simulink model "lowpasscont2"  (Simulink 8.3)
settings: Solver=ode4  StartTime=0.0  StopTime=10.24  FixedStep=dt  MaxStep=自動  MinStep=自動  RelTol=1e-3  AbsTol=自動
values from neighbouring files (symbols this model uses):
  dt = 0.01    [p217.m]    (also in p218_2.m; p223.m)
settings Model: Creator=ikko  LastModifiedBy=ikko
settings SolverCC: InitialStep=自動
settings DataIOCC: SignalLoggingName=logsOut
settings OptimizationCC: ExpressionDepthLimit=2147483647  InitFltsAndDblsToZero=on
settings DebuggingCC: SaveWithParameterizedLinksMsg=none  CheckExecutionContextPreStartOutputMsg=on  CheckExecutionContextRuntimeOutputMsg=on  SignalResolutionControl=TryResolveAllWithWarning  MultiTaskDSMMsg=warning  MultiTaskCondExecSysMsg=none  FcnCallInpInsideContextMsg=EnableAllAsWarning  StrictBusMsg=None
settings RTWCC: IncludeERTFirstTime=on
settings GRTTargetCC: TargetFcnLib=ansi_tfl_tmw.mat

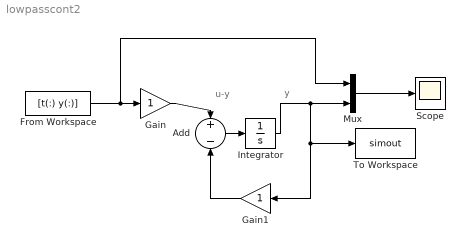
== system lowpasscont2 ==
  note: u-y
  note: y
  Add : Sum  Inputs=+-
  From Workspace : FromWorkspace  VariableName=[t(:) y(:)]  SampleTime=dt
  Gain : Gain
  Gain1 : Gain
  Integrator : Integrator
  Mux : Mux  Inputs=2
  Scope : Scope
  To Workspace : ToWorkspace  VariableName=simout  SaveFormat=Structure  SampleTime=-1
      settings: MaxDataPoints=length(t)
  wires:
  Integrator/1 -> Mux/2, To Workspace/1, Gain1/1
  Mux/1 -> Scope/1
  From Workspace/1 -> Mux/1, Gain/1
  Gain/1 -> Add/1
  Add/1 -> Integrator/1
  Gain1/1 -> Add/2
